simulink model "Robot de Parqueo"  (R2014a)
settings: Solver=ode3  SolverMode=SingleTasking  StartTime=0.0  StopTime=10.0  RelTol=1e-3
undefined symbols (not defined in the file): Normalized
libraries: legonxtlib x6
settings Model: ExtModeTrigDuration=2  Creator=david  LastModifiedBy=EDUARDO
settings OptimizationCC: OptimizeModelRefInitCode=on  LifeSpan=1
settings DebuggingCC: UnderspecifiedInitializationDetection=Classic  SolverPrmCheckMsg=none
settings HardwareCC: ProdLargestAtomicInteger=Long  ProdLargestAtomicFloat=Float  ProdEndianess=LittleEndian  ProdHWDeviceType=ARM Compatible->ARM 7
settings RTWCC: SystemTargetFile=realtime.tlc  GenerateMakefile=off  TemplateMakefile=realtime.tmf  Description=Run on Target Hardware  RTWVerbose=off  ProcessScript=realtime_make_rtw_hook
settings STFCustomTargetCC: TargetLibSuffix=.a  GenerateSampleERTMain=on  ConcurrentExecutionCompliant=off  GeneratePreprocessorConditionals=Use local settings  ERTCustomFileBanners=on  SupportNonInlinedSFcns=off  SupportVariableSizeSignals=on  MATLABClassNameForMDSCustomization=Simulink.SoftwareTarget.ERTCustomization  GRTInterface=off  SystemTargetFile=realtime.tlc
settings ERTTargetCC: CombineOutputUpdateFcns=off  SupportContinuousTime=on  SupportVariableSizeSignals=on  ExtModeTransport=2  ExtModeMexFile=ext_serial_win32_comm_no_acks_rtt  ExtModeMexArgs=0 1 9600  ERTSrcFileBannerTemplate=realtime_code_template.cgt  ERTHdrFileBannerTemplate=realtime_code_template.cgt  ERTDataSrcFileTemplate=realtime_code_template.cgt  ERTDataHdrFileTemplate=realtime_code_template.cgt  ERTCustomFileTemplate=realtime_file_process.tlc

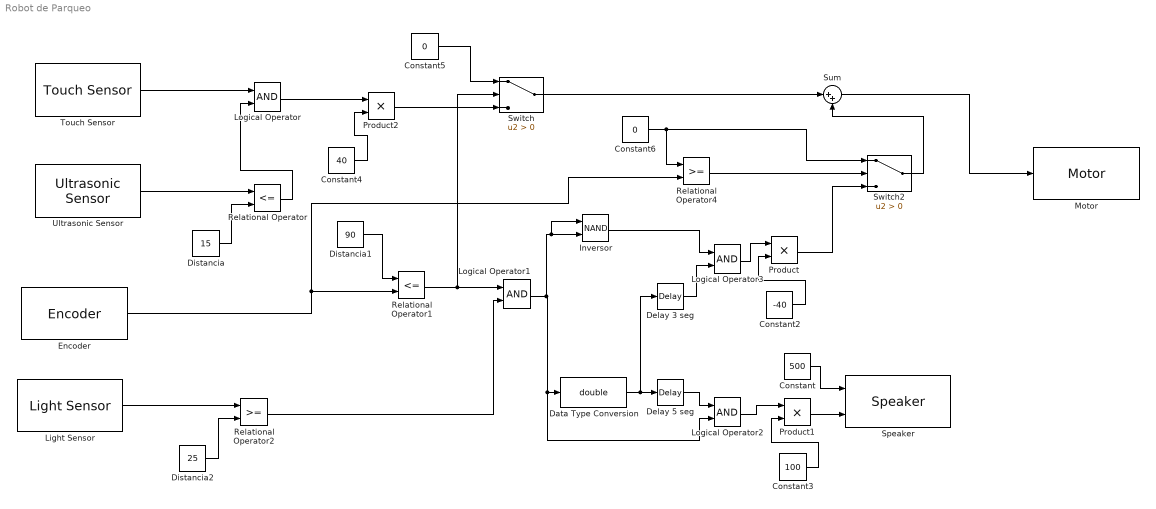
== system Robot de Parqueo ==
  Constant : Constant  Value=500
  Constant2 : Constant  Value=-40
  Constant3 : Constant  Value=100
  Constant4 : Constant  Value=40
  Constant5 : Constant  Value=0
  Constant6 : Constant  Value=0
  Data Type Conversion : DataTypeConversion  OutDataTypeStr=double
  Delay 3 seg : TransportDelay  DelayTime=3
  Delay 5 seg : TransportDelay  DelayTime=5
  Distancia : Constant  Value=15
  Distancia1 : Constant  Value=90
  Distancia2 : Constant  Value=25
  Encoder : legonxtlib/Encoder  portNumber=A  opMode=No reset  sampleTime=0.1
  Inversor : Logic  Operator=NAND  AllPortsSameDT=off  OutDataTypeStr=boolean
  Light Sensor : legonxtlib/Light Sensor  portNumber=3  outputMode=Normalized (0 -100)  lightOn=on  sampleTime=0.1
  Logical Operator : Logic  AllPortsSameDT=off  OutDataTypeStr=fixdt(0,1)
  Logical Operator1 : Logic  AllPortsSameDT=off  OutDataTypeStr=boolean
  Logical Operator2 : Logic  AllPortsSameDT=off  OutDataTypeStr=fixdt(0,1)
  Logical Operator3 : Logic  AllPortsSameDT=off  OutDataTypeStr=fixdt(0,1)
  Motor : legonxtlib/Motor  sportNumber=A  sstopAction=Brake
  Product : Product
  Product1 : Product
  Product2 : Product
  Relational Operator : RelationalOperator  Operator=<=  OutDataTypeStr=fixdt(0,1)
  Relational Operator1 : RelationalOperator  Operator=<=  OutDataTypeStr=boolean
  Relational Operator2 : RelationalOperator  OutDataTypeStr=boolean
  Relational Operator4 : RelationalOperator  OutDataTypeStr=fixdt(0,1)
  Speaker : legonxtlib/Speaker  sinputMode=Frequency and volume  sspeakerFreq=100  sspeakerVolume=50  sspeakerDuration=2000
  Sum : Sum  Inputs=|++
  Switch : Switch  Criteria=u2 > Threshold
  Switch2 : Switch  Criteria=u2 > Threshold
  Touch Sensor : legonxtlib/Touch Sensor  portNumber=1  sampleTime=0.1
  Ultrasonic Sensor : legonxtlib/Ultrasonic Sensor  PortNumber=2  sampleTime=0.1
  wires:
  Distancia1/1 -> Relational Operator1/1
  Light Sensor/1 -> Relational Operator2/1
  Distancia2/1 -> Relational Operator2/2
  Relational Operator2/1 -> Logical Operator1/2
  Product1/1 -> Speaker/2
  Constant/1 -> Speaker/1
  Delay 5 seg/1 -> Logical Operator2/1
  Relational Operator1/1 -> Switch/2, Logical Operator1/1
  Logical Operator1/1 -> Inversor/2, Inversor/1, Logical Operator2/2, Data Type Conversion/1
  Data Type Conversion/1 -> Delay 3 seg/1, Delay 5 seg/1
  Inversor/1 -> Logical Operator3/1
  Delay 3 seg/1 -> Logical Operator3/2
  Logical Operator3/1 -> Product/1
  Constant2/1 -> Product/2
  Constant3/1 -> Product1/2
  Logical Operator2/1 -> Product1/1
  Ultrasonic Sensor/1 -> Relational Operator/1
  Distancia/1 -> Relational Operator/2
  Relational Operator/1 -> Logical Operator/2
  Constant5/1 -> Switch/1
  Product2/1 -> Switch/3
  Constant4/1 -> Product2/2
  Logical Operator/1 -> Product2/1
  Touch Sensor/1 -> Logical Operator/1
  Sum/1 -> Motor/1
  Switch/1 -> Sum/1
  Product/1 -> Switch2/3
  Switch2/1 -> Sum/2
  Encoder/1 -> Relational Operator4/2, Relational Operator1/2
  Constant6/1 -> Switch2/1, Relational Operator4/1
  Relational Operator4/1 -> Switch2/2
